simulink model "vertical_dynamics_vehicle"  (R2025a)
settings: Solver=FixedStepAuto  StartTime=0.0  StopTime=T_sim  FixedStep=T_abt  RelTol=1e-3
values from neighbouring files (symbols this model uses):
  b = 1.4    [vertical_dynamics_kf.m]
  dFh = 2000    [vertical_dynamics_kf.m]
  dFv = 1500    [vertical_dynamics_kf.m]
  dPhi_0 = 0    [vertical_dynamics_kf.m]
  dR = 250    [vertical_dynamics_kf.m]
  dTheta_0 = 0    [vertical_dynamics_kf.m]
  dz1_0 = 0    [vertical_dynamics_kf.m]
  dz2_0 = 0    [vertical_dynamics_kf.m]
  dz3_0 = 0    [vertical_dynamics_kf.m]
  dz4_0 = 0    [vertical_dynamics_kf.m]
  dz5_0 = 0    [vertical_dynamics_kf.m]
  Jphi = 500    [vertical_dynamics_kf.m]
  Jtheta = 2000    [vertical_dynamics_kf.m]
  kFh = 2200    [vertical_dynamics_kf.m]
  kFv = 2500    [vertical_dynamics_kf.m]
  kR = 100000    [vertical_dynamics_kf.m]
  lh = 1.8    [vertical_dynamics_kf.m]
  lv = 1.9    [vertical_dynamics_kf.m]
  m1 = 50    [vertical_dynamics_kf.m]
  m2 = 50    [vertical_dynamics_kf.m]
  m3 = 50    [vertical_dynamics_kf.m]
  m4 = 50    [vertical_dynamics_kf.m]
  m5 = 1200    [vertical_dynamics_kf.m]
  P_0 = Q    [vertical_dynamics_kf.m]
  Phi_0 = 0    [vertical_dynamics_kf.m]
  Q = diag([sigma_z^2,sigma_z^2,sigma_z^2,sigma_z^2,sigma_z^2,sigma_phi^2,sigma_theta^2,    sigma_dz^2,sigma_dz^2,sigma_dz^2,sigma_dz^2,sigma_dz^2,sigma_dphi^2,sigma_dtheta^2 ])*T_abt^2    [vertical_dynamics_kf.m]
  R = diag([sigma_mz^2,sigma_mz^2,sigma_mz^2,sigma_mz^2,sigma_mz^2,sigma_mphi^2,sigma_mtheta^2])    [vertical_dynamics_kf.m]
  seed = randi(1000,3,1)    [vertical_dynamics_kf.m]
  sigma_dphi = 1.6    [vertical_dynamics_kf.m]
  sigma_dtheta = 1.3    [vertical_dynamics_kf.m]
  sigma_dz = 1.1    [vertical_dynamics_kf.m]
  sigma_mphi = 0.2    [vertical_dynamics_kf.m]
  sigma_mtheta = 0.1    [vertical_dynamics_kf.m]
  sigma_mz = 0.1    [vertical_dynamics_kf.m]
  sigma_phi = 1.2    [vertical_dynamics_kf.m]
  sigma_theta = 1.7    [vertical_dynamics_kf.m]
  sigma_z = 1.5    [vertical_dynamics_kf.m]
  T_abt = 0.01    [vertical_dynamics_kf.m]
  Theta_0 = 0    [vertical_dynamics_kf.m]
  x_0 = [z1_0;z2_0;z3_0;z4_0;z5_0;Phi_0;Theta_0;dz1_0;dz2_0;dz3_0;dz4_0;dz5_0;dPhi_0;dTheta_0]    [vertical_dynamics_kf.m]
  z1_0 = 0    [vertical_dynamics_kf.m]
  z2_0 = 0    [vertical_dynamics_kf.m]
  z3_0 = 0    [vertical_dynamics_kf.m]
  z4_0 = 0    [vertical_dynamics_kf.m]
  z5_0 = 0    [vertical_dynamics_kf.m]
(part 1 of 2)
settings Model: Creator=Meng Lingbing  LastModifiedBy=CelestialAurora
settings DataIOCC: ReturnWorkspaceOutputs=off
settings RTWCC: GPUComputeCapability=3.5

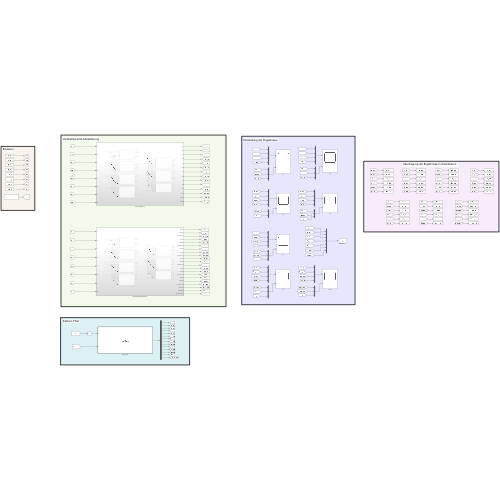
[thumbnail: Simulink's stored preview of the top-level diagram]
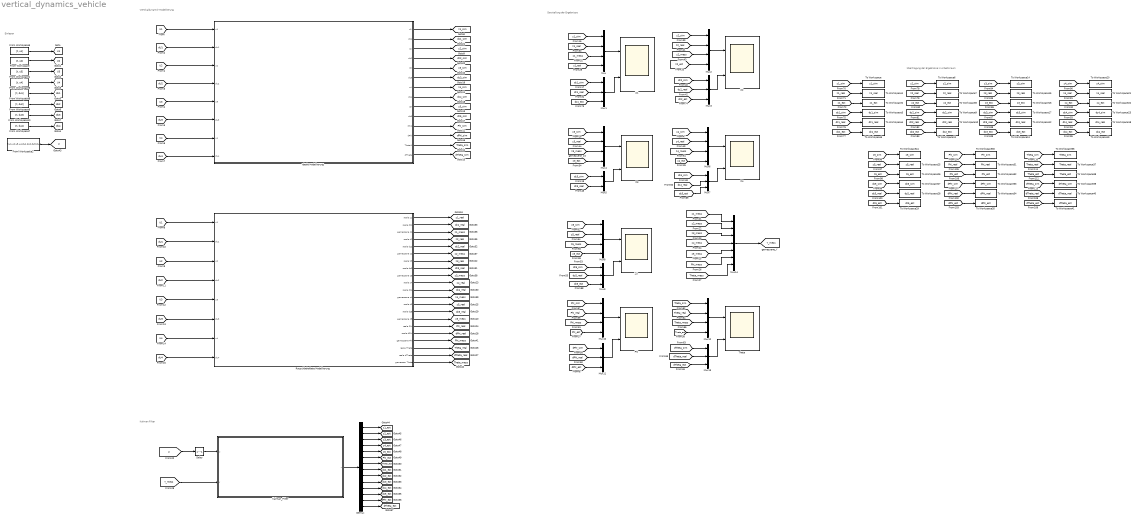
== system vertical_dynamics_vehicle ==
  note: Übertragung der Ergebnisse in Arbeitsraum
  note: Kalman Filter
  note: Einlesen
  note: Vertikaldynamik-Modellierung
  note: Darstellung der Ergebnisse
  Delay : Delay  DelayLength=1  InitialCondition=0
  Demux : Demux  Outputs=14
  From Workspace : FromWorkspace  VariableName=[t, u2]
  From Workspace1 : FromWorkspace  VariableName=[t, u3]
  From Workspace10 : FromWorkspace  VariableName=[t, du3]
  From Workspace2 : FromWorkspace  VariableName=[t,u1,u2,u3,u4,du1,du2,du3,du4]
  From Workspace5 : FromWorkspace  VariableName=[t, u1]
  From Workspace6 : FromWorkspace  VariableName=[t, u4]
  From Workspace7 : FromWorkspace  VariableName=[t, du4]
  From Workspace8 : FromWorkspace  VariableName=[t, du1]
  From Workspace9 : FromWorkspace  VariableName=[t, du2]
  Ideale Modellierung : Subsystem
  Kalman_Filter : MATLAB Function  TreatAsAtomicUnit=on
  Mux{,2,4,6,8,10,12} (7 alike) : Mux
  Mux{1,3,7,9,11,13} (6 alike) : Mux  Inputs=3
  Mux14 : Mux  Inputs=7
  Mux5 : Mux  Inputs=2
  Phi : Scope  NumInputPorts=2
      settings: Title=Phi  ActiveDisplayYMinimum=-0.7996543826921555  ActiveDisplayYMaximum=0.79993168814279936  DataLoggingVariableName=ScopeData5
  Rauschbehaftete Modellierung : Subsystem
  Theta : Scope  NumInputPorts=2
      settings: Title=Theta  ActiveDisplayYMinimum=-0.43128  ActiveDisplayYMaximum=0.39189  DataLoggingVariableName=ScopeData6
  To Workspace : ToWorkspace  VariableName=z1_sim  SampleTime=-1
      settings: Save2DSignal=2-D array (concatenate along first dimension)
  To Workspace1 : ToWorkspace  VariableName=z1_real  SampleTime=-1
      settings: Save2DSignal=2-D array (concatenate along first dimension)
  To Workspace10 : ToWorkspace  VariableName=dz2_real  SampleTime=-1
      settings: Save2DSignal=2-D array (concatenate along first dimension)
  To Workspace11 : ToWorkspace  VariableName=dz2_est  SampleTime=-1
      settings: Save2DSignal=2-D array (concatenate along first dimension)
  To Workspace12 : ToWorkspace  VariableName=dz3_real  SampleTime=-1
      settings: Save2DSignal=2-D array (concatenate along first dimension)
  To Workspace13 : ToWorkspace  VariableName=dz3_est  SampleTime=-1
      settings: Save2DSignal=2-D array (concatenate along first dimension)
  To Workspace14 : ToWorkspace  VariableName=z3_sim  SampleTime=-1
      settings: Save2DSignal=2-D array (concatenate along first dimension)
  To Workspace15 : ToWorkspace  VariableName=z3_real  SampleTime=-1
      settings: Save2DSignal=2-D array (concatenate along first dimension)
  To Workspace16 : ToWorkspace  VariableName=z3_est  SampleTime=-1
      settings: Save2DSignal=2-D array (concatenate along first dimension)
  To Workspace17 : ToWorkspace  VariableName=dz3_sim  SampleTime=-1
      settings: Save2DSignal=2-D array (concatenate along first dimension)
  To Workspace18 : ToWorkspace  VariableName=dz4_real  SampleTime=-1
      settings: Save2DSignal=2-D array (concatenate along first dimension)
  To Workspace19 : ToWorkspace  VariableName=dz4_est  SampleTime=-1
      settings: Save2DSignal=2-D array (concatenate along first dimension)
  To Workspace2 : ToWorkspace  VariableName=z1_est  SampleTime=-1
      settings: Save2DSignal=2-D array (concatenate along first dimension)
  To Workspace20 : ToWorkspace  VariableName=z4_sim  SampleTime=-1
      settings: Save2DSignal=2-D array (concatenate along first dimension)
  To Workspace21 : ToWorkspace  VariableName=z4_real  SampleTime=-1
      settings: Save2DSignal=2-D array (concatenate along first dimension)
  To Workspace22 : ToWorkspace  VariableName=z4_est  SampleTime=-1
      settings: Save2DSignal=2-D array (concatenate along first dimension)
  To Workspace23 : ToWorkspace  VariableName=dz4_sim  SampleTime=-1
      settings: Save2DSignal=2-D array (concatenate along first dimension)
  To Workspace24 : ToWorkspace  VariableName=z5_sim  SampleTime=-1
      settings: Save2DSignal=2-D array (concatenate along first dimension)
  To Workspace25 : ToWorkspace  VariableName=z5_real  SampleTime=-1
      settings: Save2DSignal=2-D array (concatenate along first dimension)
  To Workspace26 : ToWorkspace  VariableName=z5_est  SampleTime=-1
      settings: Save2DSignal=2-D array (concatenate along first dimension)
  To Workspace27 : ToWorkspace  VariableName=dz5_sim  SampleTime=-1
      settings: Save2DSignal=2-D array (concatenate along first dimension)
  To Workspace28 : ToWorkspace  VariableName=dz5_real  SampleTime=-1
      settings: Save2DSignal=2-D array (concatenate along first dimension)
  To Workspace29 : ToWorkspace  VariableName=dz5_est  SampleTime=-1
      settings: Save2DSignal=2-D array (concatenate along first dimension)
  To Workspace3 : ToWorkspace  VariableName=dz1_sim  SampleTime=-1
      settings: Save2DSignal=2-D array (concatenate along first dimension)
  To Workspace30 : ToWorkspace  VariableName=Phi_sim  SampleTime=-1
      settings: Save2DSignal=2-D array (concatenate along first dimension)
  To Workspace31 : ToWorkspace  VariableName=Phi_real  SampleTime=-1
      settings: Save2DSignal=2-D array (concatenate along first dimension)
  To Workspace32 : ToWorkspace  VariableName=Phi_est  SampleTime=-1
      settings: Save2DSignal=2-D array (concatenate along first dimension)
  To Workspace33 : ToWorkspace  VariableName=dPhi_sim  SampleTime=-1
      settings: Save2DSignal=2-D array (concatenate along first dimension)
  To Workspace34 : ToWorkspace  VariableName=dPhi_real  SampleTime=-1
      settings: Save2DSignal=2-D array (concatenate along first dimension)
  To Workspace35 : ToWorkspace  VariableName=dPhi_est  SampleTime=-1
      settings: Save2DSignal=2-D array (concatenate along first dimension)
  To Workspace36 : ToWorkspace  VariableName=Theta_sim  SampleTime=-1
      settings: Save2DSignal=2-D array (concatenate along first dimension)
  To Workspace37 : ToWorkspace  VariableName=Theta_real  SampleTime=-1
      settings: Save2DSignal=2-D array (concatenate along first dimension)
  To Workspace38 : ToWorkspace  VariableName=Theta_est  SampleTime=-1
      settings: Save2DSignal=2-D array (concatenate along first dimension)
  To Workspace39 : ToWorkspace  VariableName=dTheta_sim  SampleTime=-1
      settings: Save2DSignal=2-D array (concatenate along first dimension)
  To Workspace4 : ToWorkspace  VariableName=dz1_real  SampleTime=-1
      settings: Save2DSignal=2-D array (concatenate along first dimension)
  To Workspace40 : ToWorkspace  VariableName=dTheta_real  SampleTime=-1
      settings: Save2DSignal=2-D array (concatenate along first dimension)
  To Workspace41 : ToWorkspace  VariableName=dTheta_est  SampleTime=-1
      settings: Save2DSignal=2-D array (concatenate along first dimension)
  To Workspace5 : ToWorkspace  VariableName=dz1_est  SampleTime=-1
      settings: Save2DSignal=2-D array (concatenate along first dimension)
  To Workspace6 : ToWorkspace  VariableName=z2_sim  SampleTime=-1
      settings: Save2DSignal=2-D array (concatenate along first dimension)
  To Workspace7 : ToWorkspace  VariableName=z2_real  SampleTime=-1
      settings: Save2DSignal=2-D array (concatenate along first dimension)
  To Workspace8 : ToWorkspace  VariableName=z2_est  SampleTime=-1
      settings: Save2DSignal=2-D array (concatenate along first dimension)
  To Workspace9 : ToWorkspace  VariableName=dz2_sim  SampleTime=-1
      settings: Save2DSignal=2-D array (concatenate along first dimension)
  Z{1..5} (5 alike) : Scope  NumInputPorts=2
      Z1 settings: ActiveDisplayYMinimum=-0.48807654529336147  ActiveDisplayYMaximum=0.4265472667177741  DataLoggingVariableName=Z1  DataLoggingSaveFormat=Structure
      Z2 settings: ActiveDisplayYMinimum=-4.09102  ActiveDisplayYMaximum=3.79326
      Z3 settings: ActiveDisplayYMinimum=-4.04069  ActiveDisplayYMaximum=4.12549  DataLoggingVariableName=ScopeData2
      Z4 settings: ActiveDisplayYMinimum=-3.98296  ActiveDisplayYMaximum=4.0701  DataLoggingVariableName=ScopeData3
      Z5 settings: Title=Z5  ActiveDisplayYMinimum=-0.43929  ActiveDisplayYMaximum=0.39174  DataLoggingVariableName=ScopeData4
  tag scope: Phi_est=global, Phi_mess=global, Phi_real=global, Phi_sim=global, Theta_est=global, Theta_mess=global, Theta_real=global, Theta_sim=global, U1=global, U2=global, U3=global, U4=global, U=global, Y_mess=global, dPhi_est=global, dPhi_real=global, dPhi_sim=global, dTheta_est=global, dTheta_real=global, dTheta_sim=global, dU1=global, dU2=global, dU3=global, dU4=global, dz1_est=global, dz1_real=global, dz1_sim=global, dz2_est=global, dz2_real=global, dz2_sim=global, dz3_est=global, dz3_real=global, dz3_sim=global, dz4_est=global, dz4_real=global, dz4_sim=global, dz5_est=global, dz5_real=global, dz5_sim=global, z1_est=global, z1_mess=global, z1_real=global, z1_sim=global, z2_est=global, z2_mess=global, z2_real=global, z2_sim=global, z3_est=global, z3_mess=global, z3_real=global, z3_sim=global, z4_est=global, z4_mess=global, z4_real=global, z4_sim=global, z5_est=global, z5_mess=global, z5_real=global, z5_sim=global
  wires:
  From Workspace5/1 -> [U1]
  From Workspace/1 -> [U2]
  From Workspace1/1 -> [U3]
  From Workspace6/1 -> [U4]
  From Workspace7/1 -> [dU4]
  From Workspace8/1 -> [dU1]
  From Workspace9/1 -> [dU2]
  From Workspace10/1 -> [dU3]
  [U1] -> Ideale Modellierung/1(u1)
  [dU1] -> Ideale Modellierung/2(du1)
  [U2] -> Ideale Modellierung/3(u2)
  [dU2] -> Ideale Modellierung/4(du2)
  [U3] -> Ideale Modellierung/5(u3)
  [dU3] -> Ideale Modellierung/6(du3)
  [U4] -> Ideale Modellierung/7(u4)
  [dU4] -> Ideale Modellierung/8(du4)
  Ideale Modellierung/1(z1) -> [z1_sim]
  Ideale Modellierung/3(z2) -> [z2_sim]
  Ideale Modellierung/5(z3) -> [z3_sim]
  Ideale Modellierung/7(z4) -> [z4_sim]
  Ideale Modellierung/9(z5) -> [z5_sim]
  Ideale Modellierung/11(Phi1) -> [Phi_sim]
  Ideale Modellierung/13(Theta1) -> [Theta_sim]
  Ideale Modellierung/2(dz1) -> [dz1_sim]
  Ideale Modellierung/10(dz5) -> [dz5_sim]
  Ideale Modellierung/8(dz4) -> [dz4_sim]
  Ideale Modellierung/6(dz3) -> [dz3_sim]
  Ideale Modellierung/4(dz2) -> [dz2_sim]
  Ideale Modellierung/12(dPhi) -> [dPhi_sim]
  Ideale Modellierung/14(dTheta) -> [dTheta_sim]
  Rauschbehaftete Modellierung/17(reale dPhi) -> [dPhi_real]
  Rauschbehaftete Modellierung/1(reale z1) -> [z1_real]
  [dU3] -> Rauschbehaftete Modellierung/6(du3)
  [dU4] -> Rauschbehaftete Modellierung/8(du4)
  Rauschbehaftete Modellierung/13(reale z5) -> [z5_real]
  Rauschbehaftete Modellierung/7(reale z3) -> [z3_real]
  Rauschbehaftete Modellierung/19(reale Theta) -> [Theta_real]
  Rauschbehaftete Modellierung/10(reale z4) -> [z4_real]
  Rauschbehaftete Modellierung/16(reale Phi) -> [Phi_real]
  [U3] -> Rauschbehaftete Modellierung/5(u3)
  [dU2] -> Rauschbehaftete Modellierung/4(du2)
  Rauschbehaftete Modellierung/4(reale z2) -> [z2_real]
  [U1] -> Rauschbehaftete Modellierung/1(u1)
  [dU1] -> Rauschbehaftete Modellierung/2(du1)
  Rauschbehaftete Modellierung/5(reale dz2) -> [dz2_real]
  Rauschbehaftete Modellierung/8(reale dz3) -> [dz3_real]
  Rauschbehaftete Modellierung/14(reale dz5) -> [dz5_real]
  Rauschbehaftete Modellierung/11(reale dz4) -> [dz4_real]
  Rauschbehaftete Modellierung/20(reale dTheta) -> [dTheta_real]
  [U2] -> Rauschbehaftete Modellierung/3(u2)
  [U4] -> Rauschbehaftete Modellierung/7(u4)
  Rauschbehaftete Modellierung/2(reale dz1) -> [dz1_real]
  Rauschbehaftete Modellierung/3(gemessene z1) -> [z1_mess]
  Rauschbehaftete Modellierung/6(gemessene z2) -> [z2_mess]
  Rauschbehaftete Modellierung/9(gemessene z3) -> [z3_mess]
  Rauschbehaftete Modellierung/12(gemessene z4) -> [z4_mess]
  Rauschbehaftete Modellierung/15(gemessene z5) -> [z5_mess]
  Rauschbehaftete Modellierung/18(gemessene Phi) -> [Phi_mess]
  Rauschbehaftete Modellierung/21(gemessen Theta) -> [Theta_mess]
  [z1_sim] -> Mux/1
  [z1_real] -> Mux/2
  [z1_mess] -> Mux/3
  [dz1_sim] -> Mux1/1
  [dz1_real] -> Mux1/2
  Mux/1 -> Z1/1
  Mux1/1 -> Z1/2
  [z2_sim] -> Mux2/1
  [dz2_real] -> Mux3/2
  [dz2_sim] -> Mux3/1
  Mux2/1 -> Z2/1
  [z2_real] -> Mux2/2
  Mux3/1 -> Z2/2
  [z2_mess] -> Mux2/3
  [z3_sim] -> Mux4/1
  [dz3_real] -> Mux5/2
  [dz3_sim] -> Mux5/1
  Mux4/1 -> Z3/1
  [z3_real] -> Mux4/2
  Mux5/1 -> Z3/2
  [z3_mess] -> Mux4/3
  [z4_real] -> Mux6/2
  Mux6/1 -> Z4/1
  [z4_mess] -> Mux6/3
  [dz4_sim] -> Mux7/1
  [dz4_real] -> Mux7/2
  [z4_sim] -> Mux6/1
  Mux7/1 -> Z4/2
  Mux9/1 -> Z5/2
  [z5_real] -> Mux8/2
  Mux8/1 -> Z5/1
  [z5_sim] -> Mux8/1
  [dz5_sim] -> Mux9/1
  [z5_mess] -> Mux8/3
  [dz5_real] -> Mux9/2
  Mux11/1 -> Phi/2
  [Phi_real] -> Mux10/2
  Mux10/1 -> Phi/1
  [Phi_sim] -> Mux10/1
  [dPhi_sim] -> Mux11/1
  [Phi_mess] -> Mux10/3
  [dPhi_real] -> Mux11/2
  Mux13/1 -> Theta/2
  [Theta_real] -> Mux12/2
  Mux12/1 -> Theta/1
  [Theta_sim] -> Mux12/1
  [dTheta_sim] -> Mux13/1
  [Theta_mess] -> Mux12/3
  [dTheta_real] -> Mux13/2
  From Workspace2/1 -> [U]
  [U] -> Delay/1
  [z4_mess] -> Mux14/4
  [z3_mess] -> Mux14/3
  [z2_mess] -> Mux14/2
  [z1_mess] -> Mux14/1
  [z5_mess] -> Mux14/5
  [Phi_mess] -> Mux14/6
  [Theta_mess] -> Mux14/7
  Mux14/1 -> [Y_mess]
  [Y_mess] -> Kalman_Filter/2(y)
  Kalman_Filter/1(x) -> Demux/1
  Demux/1 -> [z1_est]
  Demux/2 -> [z2_est]
  Demux/3 -> [z3_est]
  Demux/4 -> [z4_est]
  Demux/5 -> [z5_est]
  Demux/6 -> [Phi_est]
  Demux/7 -> [Theta_est]
  Demux/8 -> [dz1_est]
  Demux/9 -> [dz2_est]
  Demux/10 -> [dz3_est]
  Demux/11 -> [dz4_est]
  Demux/12 -> [dz5_est]
  Demux/13 -> [dPhi_est]
  Demux/14 -> [dTheta_est]
  Delay/1 -> Kalman_Filter/1(u)
  [z1_est] -> Mux/4
  [z2_est] -> Mux2/4
  [z3_est] -> Mux4/4
  [z4_est] -> Mux6/4
  [z5_est] -> Mux8/4
  [Phi_est] -> Mux10/4
  [Theta_est] -> Mux12/4
  [dTheta_est] -> Mux13/3
  [dPhi_est] -> Mux11/3
  [dz5_est] -> Mux9/3
  [dz5_est] -> Mux7/3
  [dz1_est] -> Mux1/3
  [dz2_est] -> Mux3/3
  [z1_sim] -> To Workspace/1
  [z1_real] -> To Workspace1/1
  [z1_est] -> To Workspace2/1
  [dz1_est] -> To Workspace5/1
  [dz1_real] -> To Workspace4/1
  [dz1_sim] -> To Workspace3/1
  [dz2_est] -> To Workspace11/1
  [dz2_sim] -> To Workspace9/1
  [z2_real] -> To Workspace7/1
  [dz2_real] -> To Workspace10/1
  [z2_sim] -> To Workspace6/1
  [z2_est] -> To Workspace8/1
  [z3_est] -> To Workspace16/1
  [z3_real] -> To Workspace15/1
  [dz3_est] -> To Workspace13/1
  [z3_sim] -> To Workspace14/1
  [dz3_real] -> To Workspace12/1
  [dz3_sim] -> To Workspace17/1
  [dz4_sim] -> To Workspace23/1
  [dz4_real] -> To Workspace18/1
  [z4_sim] -> To Workspace20/1
  [dz4_est] -> To Workspace19/1
  [z4_real] -> To Workspace21/1
  [z4_est] -> To Workspace22/1
  [dz5_est] -> To Workspace29/1
  [dz5_sim] -> To Workspace27/1
  [z5_real] -> To Workspace25/1
  [dz5_real] -> To Workspace28/1
  [z5_sim] -> To Workspace24/1
  [z5_est] -> To Workspace26/1
  [Phi_sim] -> To Workspace30/1
  [dPhi_sim] -> To Workspace33/1
  [Phi_est] -> To Workspace32/1
  [dPhi_real] -> To Workspace34/1
  [Phi_real] -> To Workspace31/1
  [dPhi_est] -> To Workspace35/1
  [Theta_real] -> To Workspace37/1
  [dTheta_est] -> To Workspace41/1
  [dTheta_sim] -> To Workspace39/1
  [dTheta_real] -> To Workspace40/1
  [Theta_est] -> To Workspace38/1
  [Theta_sim] -> To Workspace36/1

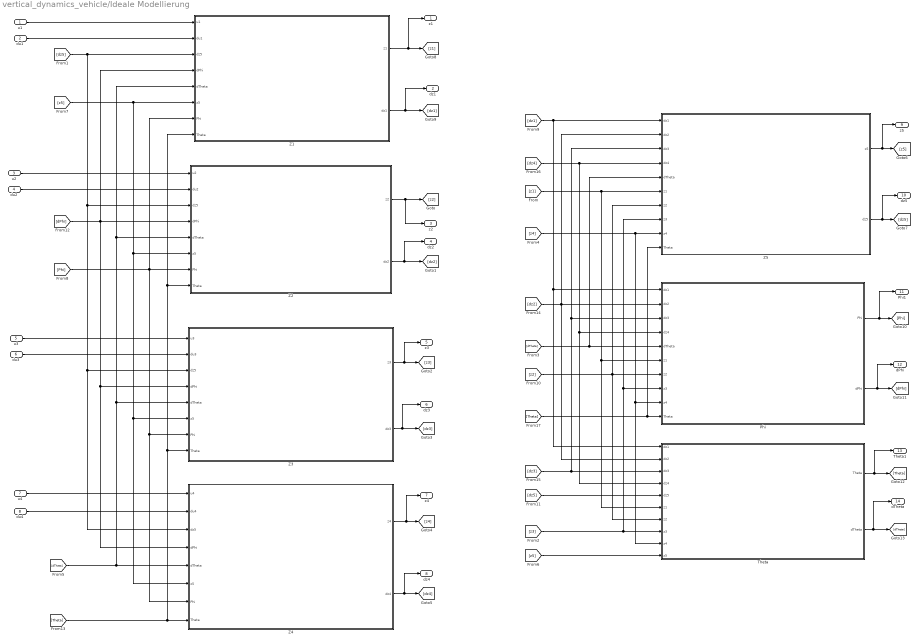
== system vertical_dynamics_vehicle/Ideale Modellierung ==
  u1 : Inport
  du1 : Inport  Port=2
  u2 : Inport  Port=3
  du2 : Inport  Port=4
  u3 : Inport  Port=5
  du3 : Inport  Port=6
  u4 : Inport  Port=7
  du4 : Inport  Port=8
  Phi : Subsystem
  Theta : Subsystem
  Z1 : Subsystem
  Z2 : Subsystem
  Z3 : Subsystem
  Z4 : Subsystem
  Z5 : Subsystem
  z1 : Outport
  dz1 : Outport  Port=2
  z2 : Outport  Port=3
  dz2 : Outport  Port=4
  z3 : Outport  Port=5
  dz3 : Outport  Port=6
  z4 : Outport  Port=7
  dz4 : Outport  Port=8
  z5 : Outport  Port=9
  dz5 : Outport  Port=10
  Phi1 : Outport  Port=11
  dPhi : Outport  Port=12
  Theta1 : Outport  Port=13
  dTheta : Outport  Port=14
  wires:
  Theta/1(Theta) -> Theta1/1, [Theta]
  Z1/1(z1) -> z1/1, [z1]
  Z1/2(dz1) -> dz1/1, [dz1]
  Z2/1(z2) -> z2/1, [z2]
  Z5/1(z5) -> [z5], z5/1
  Phi/1(Phi) -> [Phi], Phi1/1
  u1/1 -> Z1/1(u1)
  u4/1 -> Z4/1(u4)
  du4/1 -> Z4/2(du4)
  du1/1 -> Z1/2(du1)
  u2/1 -> Z2/1(u2)
  du2/1 -> Z2/2(du2)
  du3/1 -> Z3/2(du3)
  u3/1 -> Z3/1(u3)
  Z2/2(dz2) -> dz2/1, [dz2]
  Z3/1(z3) -> z3/1, [z3]
  Z3/2(dz3) -> dz3/1, [dz3]
  Z4/1(z4) -> [z4], z4/1
  Z4/2(dz4) -> dz4/1, [dz4]
  Z5/2(dz5) -> [dz5], dz5/1
  Phi/2(dPhi) -> dPhi/1, [dPhi]
  Theta/2(dTheta) -> dTheta/1, [dTheta]
  [z1] -> Z5/6(z1), Phi/6(z1), Theta/6(z1)
  [dTheta] -> Phi/5(dTheta), Z5/5(dTheta)
  [dTheta] -> Z4/5(dTheta), Z3/5(dTheta), Z2/5(dTheta), Z1/5(dTheta)
  [dz1] -> Z5/1(dz1), Phi/1(dz1), Theta/1(dz1)
  [z2] -> Phi/7(z2), Theta/7(z2), Z5/7(z2)
  [z3] -> Phi/8(z3), Z5/8(z3), Theta/8(z3)
  [dz5] -> Z1/3(dz5), Z4/3(dz5), Z3/3(dz5), Z2/3(dz5)
  [dz5] -> Theta/5(dz5)
  [dPhi] -> Z2/4(dPhi), Z3/4(dPhi), Z4/4(dPhi), Z1/4(dPhi)
  [z5] -> Z1/6(z5), Z2/6(z5), Z3/6(z5), Z4/6(z5)
  [Phi] -> Z3/7(Phi), Z4/7(Phi), Z1/7(Phi), Z2/7(Phi)
  [Theta] -> Z4/8(Theta), Z3/8(Theta), Z2/8(Theta), Z1/8(Theta)
  [dz2] -> Z5/2(dz2), Theta/2(dz2), Phi/2(dz2)
  [dz3] -> Theta/3(dz3), Phi/3(dz3), Z5/3(dz3)
  [dz4] -> Z5/4(dz4), Phi/4(dz4), Theta/4(dz4)
  [z4] -> Z5/9(z4), Phi/9(z4), Theta/9(z4)
  [Theta] -> Phi/10(Theta), Z5/10(Theta)
  [z5] -> Theta/10(z5)

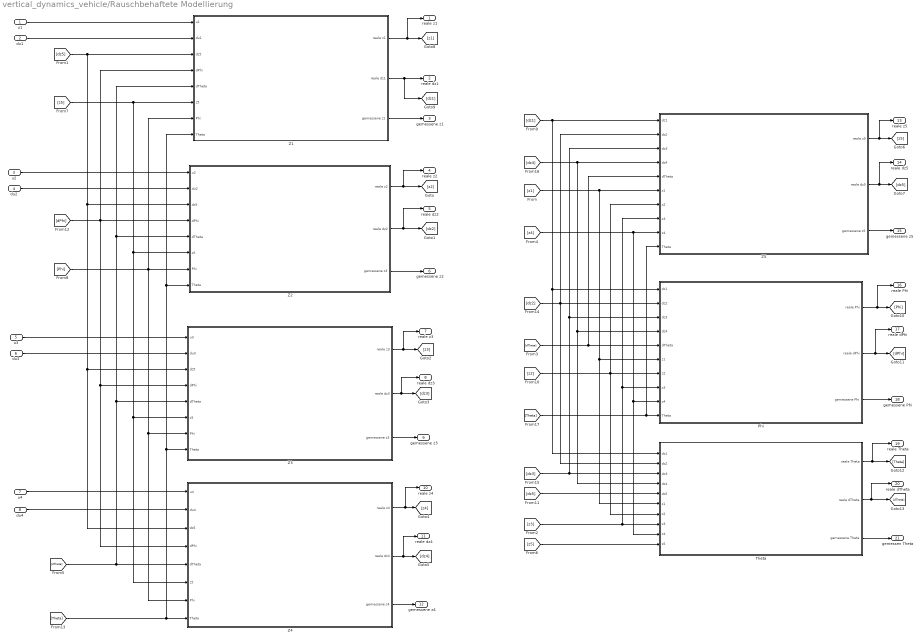
== system vertical_dynamics_vehicle/Rauschbehaftete Modellierung ==
  u1 : Inport
  du1 : Inport  Port=2
  u2 : Inport  Port=3
  du2 : Inport  Port=4
  u3 : Inport  Port=5
  du3 : Inport  Port=6
  u4 : Inport  Port=7
  du4 : Inport  Port=8
  Phi : Subsystem
  Theta : Subsystem
  Z1 : Subsystem
  Z2 : Subsystem
  Z3 : Subsystem
  Z4 : Subsystem
  Z5 : Subsystem
  reale z1 : Outport
  reale dz1 : Outport  Port=2
  gemessene z1 : Outport  Port=3
  reale z2 : Outport  Port=4
  reale dz2 : Outport  Port=5
  gemessene z2 : Outport  Port=6
  reale z3 : Outport  Port=7
  reale dz3 : Outport  Port=8
  gemessene z3 : Outport  Port=9
  reale z4 : Outport  Port=10
  reale dz4 : Outport  Port=11
  gemessene z4 : Outport  Port=12
  reale z5 : Outport  Port=13
  reale dz5 : Outport  Port=14
  gemessene z5 : Outport  Port=15
  reale Phi : Outport  Port=16
  reale dPhi : Outport  Port=17
  gemessene Phi : Outport  Port=18
  reale Theta : Outport  Port=19
  reale dTheta : Outport  Port=20
  gemessen Theta : Outport  Port=21
  wires:
  Theta/1(reale Theta) -> [Theta], reale Theta/1
  Z1/1(reale z1) -> [z1], reale z1/1
  Z1/2(reale dz1) -> [dz1], reale dz1/1
  Z2/1(reale z2) -> [z2], reale z2/1
  Z5/1(reale z5) -> [z5], reale z5/1
  Phi/1(reale Phi) -> [Phi], reale Phi/1
  u1/1 -> Z1/1(u1)
  u4/1 -> Z4/1(u4)
  du4/1 -> Z4/2(du4)
  du1/1 -> Z1/2(du1)
  u2/1 -> Z2/1(u2)
  du2/1 -> Z2/2(du2)
  du3/1 -> Z3/2(du3)
  u3/1 -> Z3/1(u3)
  Z2/2(reale dz2) -> [dz2], reale dz2/1
  Z3/1(reale z3) -> [z3], reale z3/1
  Z3/2(reale dz3) -> [dz3], reale dz3/1
  Z4/1(reale z4) -> [z4], reale z4/1
  Z4/2(reale dz4) -> [dz4], reale dz4/1
  Z5/2(reale dz5) -> [dz5], reale dz5/1
  Phi/2(reale dPhi) -> [dPhi], reale dPhi/1
  Theta/2(reale dTheta) -> [dTheta], reale dTheta/1
  [z1] -> Z5/6(z1), Phi/6(z1), Theta/6(z1)
  [dTheta] -> Phi/5(dTheta), Z5/5(dTheta)
  [dTheta] -> Z4/5(dTheta), Z3/5(dTheta), Z2/5(dTheta), Z1/5(dTheta)
  [dz1] -> Z5/1(dz1), Phi/1(dz1), Theta/1(dz1)
  [z2] -> Phi/7(z2), Theta/7(z2), Z5/7(z2)
  [z3] -> Theta/8(z3), Phi/8(z3), Z5/8(z3)
  [dz5] -> Z1/3(dz5), Z4/3(dz5), Z3/3(dz5), Z2/3(dz5)
  [dz5] -> Theta/5(dz5)
  [dPhi] -> Z2/4(dPhi), Z3/4(dPhi), Z4/4(dPhi), Z1/4(dPhi)
  [z5] -> Z1/6(z5), Z2/6(z5), Z3/6(z5), Z4/6(z5)
  [Phi] -> Z3/7(Phi), Z4/7(Phi), Z1/7(Phi), Z2/7(Phi)
  [Theta] -> Z4/8(Theta), Z3/8(Theta), Z2/8(Theta), Z1/8(Theta)
  [dz2] -> Z5/2(dz2), Theta/2(dz2), Phi/2(dz2)
  [dz3] -> Theta/3(dz3), Phi/3(dz3), Z5/3(dz3)
  [dz4] -> Z5/4(dz4), Phi/4(dz4), Theta/4(dz4)
  [z4] -> Z5/9(z4), Phi/9(z4), Theta/9(z4)
  [Theta] -> Phi/10(Theta), Z5/10(Theta)
  [z5] -> Theta/10(z5)
  Z1/3(gemessene z1) -> gemessene z1/1
  Z2/3(gemessene z3) -> gemessene z2/1
  Z3/3(gemessene z3) -> gemessene z3/1
  Z4/3(gemessene z4) -> gemessene z4/1
  Z5/3(gemessene z5) -> gemessene z5/1
  Phi/3(gemessene Phi) -> gemessene Phi/1
  Theta/3(gemessene Theta) -> gemessen Theta/1

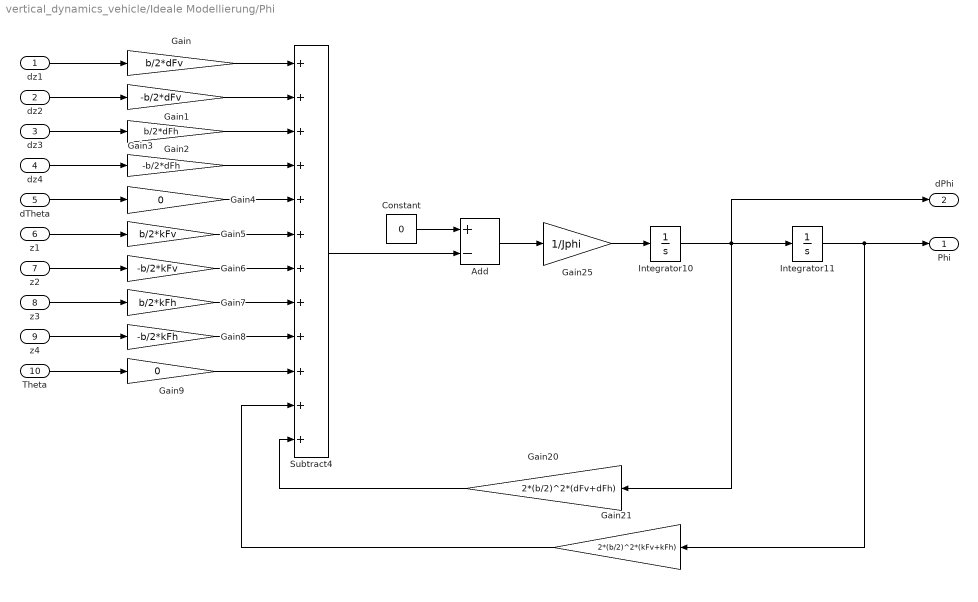
== system vertical_dynamics_vehicle/Ideale Modellierung/Phi ==
  dz1 : Inport
  dz2 : Inport  Port=2
  dz3 : Inport  Port=3
  dz4 : Inport  Port=4
  dTheta : Inport  Port=5
  z1 : Inport  Port=6
  z2 : Inport  Port=7
  z3 : Inport  Port=8
  z4 : Inport  Port=9
  Theta : Inport  Port=10
  Add : Sum  Inputs=+-
  Constant : Constant  Value=0
  Gain : Gain  Gain=b/2*dFv
  Gain1 : Gain  Gain=-b/2*dFv
  Gain2 : Gain  Gain=b/2*dFh
  Gain20 : Gain  Gain=2*(b/2)^2*(dFv+dFh)
  Gain21 : Gain  Gain=2*(b/2)^2*(kFv+kFh)
  Gain25 : Gain  Gain=1/Jphi
  Gain3 : Gain  Gain=-b/2*dFh
  Gain4 : Gain  Gain=0
  Gain5 : Gain  Gain=b/2*kFv
  Gain6 : Gain  Gain=-b/2*kFv
  Gain7 : Gain  Gain=b/2*kFh
  Gain8 : Gain  Gain=-b/2*kFh
  Gain9 : Gain  Gain=0
  Integrator10 : Integrator  InitialCondition=dPhi_0
  Integrator11 : Integrator  InitialCondition=Phi_0
  Subtract4 : Sum  Inputs=++++++++++++
  Phi : Outport
  dPhi : Outport  Port=2
  wires:
  Integrator11/1 -> Phi/1, Gain21/1
  Integrator10/1 -> Integrator11/1, dPhi/1, Gain20/1
  Gain25/1 -> Integrator10/1
  dz1/1 -> Gain/1
  Gain2/1 -> Subtract4/3
  z1/1 -> Gain5/1
  Gain9/1 -> Subtract4/10
  z3/1 -> Gain7/1
  Theta/1 -> Gain9/1
  Gain4/1 -> Subtract4/5
  Gain1/1 -> Subtract4/2
  dz2/1 -> Gain1/1
  Gain8/1 -> Subtract4/9
  dTheta/1 -> Gain4/1
  z4/1 -> Gain8/1
  Gain5/1 -> Subtract4/6
  Gain/1 -> Subtract4/1
  Gain6/1 -> Subtract4/7
  z2/1 -> Gain6/1
  dz4/1 -> Gain3/1
  Gain3/1 -> Subtract4/4
  Gain7/1 -> Subtract4/8
  dz3/1 -> Gain2/1
  Gain20/1 -> Subtract4/12
  Gain21/1 -> Subtract4/11
  Constant/1 -> Add/1
  Add/1 -> Gain25/1
  Subtract4/1 -> Add/2

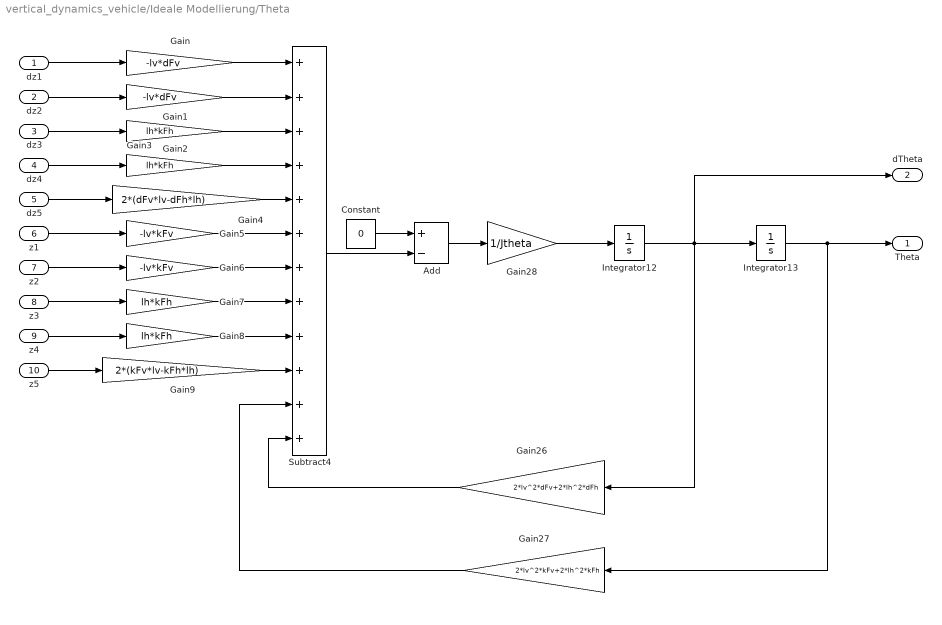
== system vertical_dynamics_vehicle/Ideale Modellierung/Theta ==
  dz1 : Inport
  dz2 : Inport  Port=2
  dz3 : Inport  Port=3
  dz4 : Inport  Port=4
  dz5 : Inport  Port=5
  z1 : Inport  Port=6
  z2 : Inport  Port=7
  z3 : Inport  Port=8
  z4 : Inport  Port=9
  z5 : Inport  Port=10
  Add : Sum  Inputs=+-
  Constant : Constant  Value=0
  Gain : Gain  Gain=-lv*dFv
  Gain1 : Gain  Gain=-lv*dFv
  Gain{2..3,7..8} (4 alike) : Gain  Gain=lh*kFh
  Gain26 : Gain  Gain=2*lv^2*dFv+2*lh^2*dFh
  Gain27 : Gain  Gain=2*lv^2*kFv+2*lh^2*kFh
  Gain28 : Gain  Gain=1/Jtheta
  Gain4 : Gain  Gain=2*(dFv*lv-dFh*lh)
  Gain5 : Gain  Gain=-lv*kFv
  Gain6 : Gain  Gain=-lv*kFv
  Gain9 : Gain  Gain=2*(kFv*lv-kFh*lh)
  Integrator12 : Integrator  InitialCondition=dTheta_0
  Integrator13 : Integrator  InitialCondition=Theta_0
  Subtract4 : Sum  Inputs=++++++++++++
  Theta : Outport
  dTheta : Outport  Port=2
  wires:
  Integrator12/1 -> Integrator13/1, dTheta/1, Gain26/1
  Integrator13/1 -> Theta/1, Gain27/1
  Gain28/1 -> Integrator12/1
  dz4/1 -> Gain3/1
  dz3/1 -> Gain2/1
  Gain7/1 -> Subtract4/8
  Gain3/1 -> Subtract4/4
  Gain/1 -> Subtract4/1
  Gain5/1 -> Subtract4/6
  dz5/1 -> Gain4/1
  Gain6/1 -> Subtract4/7
  Gain4/1 -> Subtract4/5
  Gain1/1 -> Subtract4/2
  dz2/1 -> Gain1/1
  z5/1 -> Gain9/1
  z3/1 -> Gain7/1
  dz1/1 -> Gain/1
  Gain8/1 -> Subtract4/9
  Gain9/1 -> Subtract4/10
  z1/1 -> Gain5/1
  Gain2/1 -> Subtract4/3
  z4/1 -> Gain8/1
  z2/1 -> Gain6/1
  Gain26/1 -> Subtract4/12
  Gain27/1 -> Subtract4/11
  Subtract4/1 -> Add/2
  Add/1 -> Gain28/1
  Constant/1 -> Add/1

== system vertical_dynamics_vehicle/Ideale Modellierung/Z1 ==
  u1 : Inport
  du1 : Inport  Port=2
  dz5 : Inport  Port=3
  dPhi : Inport  Port=4
  dTheta : Inport  Port=5
  z5 : Inport  Port=6
  Phi : Inport  Port=7
  Theta : Inport  Port=8
  Add : Sum
  Add1 : Sum  Inputs=8
  Add2 : Sum  Inputs=+-
  Gain : Gain  Gain=kR
  Gain1 : Gain  Gain=dR
  Gain2 : Gain  Gain=dR+dFv
  Gain29 : Gain  Gain=-dFv
  Gain3 : Gain  Gain=kR+kFv
  Gain30 : Gain  Gain=b/2*dFv
  Gain32 : Gain  Gain=-kFv
  Gain33 : Gain  Gain=b/2*kFv
  Gain34 : Gain  Gain=-lv*dFv
  Gain4 : Gain  Gain=1/m1
  Gain5 : Gain  Gain=-lv*kFv
  Integrator : Integrator  InitialCondition=dz1_0
  Integrator1 : Integrator  InitialCondition=z1_0
  z1 : Outport
  dz1 : Outport  Port=2
  wires:
  Add2/1 -> Gain4/1
  Gain1/1 -> Add/2
  Integrator/1 -> Integrator1/1, dz1/1, Gain2/1
  Gain2/1 -> Add1/1
  Add/1 -> Add2/1
  Gain/1 -> Add/1
  Gain4/1 -> Integrator/1
  Phi/1 -> Gain33/1
  Gain34/1 -> Add1/7
  Gain32/1 -> Add1/5
  Gain3/1 -> Add1/2
  Gain33/1 -> Add1/6
  u1/1 -> Gain/1
  du1/1 -> Gain1/1
  dTheta/1 -> Gain34/1
  z5/1 -> Gain32/1
  dz5/1 -> Gain29/1
  Gain29/1 -> Add1/3
  Add1/1 -> Add2/2
  Gain30/1 -> Add1/4
  dPhi/1 -> Gain30/1
  Theta/1 -> Gain5/1
  Gain5/1 -> Add1/8
  Integrator1/1 -> Gain3/1, z1/1

== system vertical_dynamics_vehicle/Ideale Modellierung/Z2 ==
  u2 : Inport
  du2 : Inport  Port=2
  dz5 : Inport  Port=3
  dPhi : Inport  Port=4
  dTheta : Inport  Port=5
  z5 : Inport  Port=6
  Phi : Inport  Port=7
  Theta : Inport  Port=8
  Add : Sum  Inputs=+-
  Add1 : Sum
  Add2 : Sum  Inputs=8
  Gain1 : Gain  Gain=-lv*kFv
  Gain29 : Gain  Gain=-dFv
  Gain30 : Gain  Gain=-b/2*dFv
  Gain32 : Gain  Gain=-kFv
  Gain33 : Gain  Gain=-b/2*kFv
  Gain34 : Gain  Gain=-lv*dFv
  Gain5 : Gain  Gain=kR
  Gain6 : Gain  Gain=dR
  Gain7 : Gain  Gain=dR+dFv
  Gain8 : Gain  Gain=kR+kFv
  Gain9 : Gain  Gain=1/m2
  Integrator2 : Integrator  InitialCondition=dz2_0
  Integrator3 : Integrator  InitialCondition=z2_0
  z2 : Outport
  dz2 : Outport  Port=2
  wires:
  Integrator2/1 -> Integrator3/1, dz2/1, Gain7/1
  Gain5/1 -> Add1/1
  du2/1 -> Gain6/1
  Integrator3/1 -> z2/1, Gain8/1
  u2/1 -> Gain5/1
  Gain9/1 -> Integrator2/1
  Gain6/1 -> Add1/2
  Gain30/1 -> Add2/4
  Gain1/1 -> Add2/8
  Theta/1 -> Gain1/1
  dPhi/1 -> Gain30/1
  Gain29/1 -> Add2/3
  Gain8/1 -> Add2/2
  Gain34/1 -> Add2/7
  dz5/1 -> Gain29/1
  Add2/1 -> Add/2
  dTheta/1 -> Gain34/1
  Gain32/1 -> Add2/5
  z5/1 -> Gain32/1
  Gain33/1 -> Add2/6
  Gain7/1 -> Add2/1
  Phi/1 -> Gain33/1
  Add1/1 -> Add/1
  Add/1 -> Gain9/1

== system vertical_dynamics_vehicle/Ideale Modellierung/Z3 ==
  u3 : Inport
  du3 : Inport  Port=2
  dz5 : Inport  Port=3
  dPhi : Inport  Port=4
  dTheta : Inport  Port=5
  z5 : Inport  Port=6
  Phi : Inport  Port=7
  Theta : Inport  Port=8
  Add1 : Sum  Inputs=8
  Add2 : Sum
  Gain1 : Gain  Gain=lh*kFh
  Gain10 : Gain  Gain=kR
  Gain11 : Gain  Gain=dR
  Gain12 : Gain  Gain=dR+dFh
  Gain13 : Gain  Gain=kR+kFh
  Gain14 : Gain  Gain=1/m3
  Gain29 : Gain  Gain=-dFh
  Gain30 : Gain  Gain=b/2*dFh
  Gain32 : Gain  Gain=-kFh
  Gain33 : Gain  Gain=b/2*kFh
  Gain34 : Gain  Gain=lh*dFh
  Integrator4 : Integrator  InitialCondition=dz3_0
  Integrator5 : Integrator  InitialCondition=z3_0
  Subtract2 : Sum  Inputs=+-
  z3 : Outport
  dz3 : Outport  Port=2
  wires:
  Gain10/1 -> Add2/1
  Add2/1 -> Subtract2/1
  Integrator4/1 -> Integrator5/1, dz3/1, Gain12/1
  Integrator5/1 -> z3/1, Gain13/1
  Gain11/1 -> Add2/2
  Gain14/1 -> Integrator4/1
  Subtract2/1 -> Gain14/1
  du3/1 -> Gain11/1
  u3/1 -> Gain10/1
  Add1/1 -> Subtract2/2
  Gain34/1 -> Add1/5
  Gain32/1 -> Add1/6
  dz5/1 -> Gain29/1
  dPhi/1 -> Gain30/1
  Theta/1 -> Gain1/1
  Gain29/1 -> Add1/3
  Gain30/1 -> Add1/4
  Gain33/1 -> Add1/7
  Gain1/1 -> Add1/8
  Gain12/1 -> Add1/1
  Gain13/1 -> Add1/2
  Phi/1 -> Gain33/1
  z5/1 -> Gain32/1
  dTheta/1 -> Gain34/1

== system vertical_dynamics_vehicle/Ideale Modellierung/Z4 ==
  u4 : Inport
  du4 : Inport  Port=2
  dz5 : Inport  Port=3
  dPhi : Inport  Port=4
  dTheta : Inport  Port=5
  z5 : Inport  Port=6
  Phi : Inport  Port=7
  Theta : Inport  Port=8
  Add1 : Sum  Inputs=8
  Add3 : Sum
  Gain1 : Gain  Gain=lh*kFh
  Gain15 : Gain  Gain=kR
  Gain16 : Gain  Gain=dR
  Gain17 : Gain  Gain=dR+dFh
  Gain18 : Gain  Gain=kR+kFh
  Gain19 : Gain  Gain=1/m4
  Gain29 : Gain  Gain=-dFh
  Gain30 : Gain  Gain=-b/2*dFh
  Gain32 : Gain  Gain=-kFh
  Gain33 : Gain  Gain=-b/2*kFh
  Gain34 : Gain  Gain=lh*dFh
  Integrator6 : Integrator  InitialCondition=dz4_0
  Integrator7 : Integrator  InitialCondition=z4_0
  Subtract3 : Sum  Inputs=+-
  z4 : Outport
  dz4 : Outport  Port=2
  wires:
  Gain16/1 -> Add3/2
  Gain17/1 -> Add1/1
  Gain15/1 -> Add3/1
  Gain19/1 -> Integrator6/1
  Add3/1 -> Subtract3/1
  Integrator7/1 -> z4/1, Gain18/1
  Integrator6/1 -> dz4/1, Gain17/1, Integrator7/1
  Subtract3/1 -> Gain19/1
  du4/1 -> Gain16/1
  u4/1 -> Gain15/1
  Add1/1 -> Subtract3/2
  Phi/1 -> Gain33/1
  z5/1 -> Gain32/1
  dTheta/1 -> Gain34/1
  Gain33/1 -> Add1/7
  dz5/1 -> Gain29/1
  Gain32/1 -> Add1/6
  Gain34/1 -> Add1/5
  Gain29/1 -> Add1/3
  Gain1/1 -> Add1/8
  dPhi/1 -> Gain30/1
  Theta/1 -> Gain1/1
  Gain30/1 -> Add1/4
  Gain18/1 -> Add1/2

== system vertical_dynamics_vehicle/Ideale Modellierung/Z5 ==
  dz1 : Inport
  dz2 : Inport  Port=2
  dz3 : Inport  Port=3
  dz4 : Inport  Port=4
  dTheta : Inport  Port=5
  z1 : Inport  Port=6
  z2 : Inport  Port=7
  z3 : Inport  Port=8
  z4 : Inport  Port=9
  Theta : Inport  Port=10
  Add : Sum  Inputs=+-
  Constant : Constant  Value=0
  Gain : Gain  Gain=-dFv
  Gain1 : Gain  Gain=-dFv
  Gain2 : Gain  Gain=-dFh
  Gain22 : Gain  Gain=2*dFv+2*dFh
  Gain23 : Gain  Gain=2*kFv+2*kFh
  Gain24 : Gain  Gain=1/m5
  Gain3 : Gain  Gain=-dFh
  Gain4 : Gain  Gain=2*(dFv*lv-dFh*lh)
  Gain5 : Gain  Gain=-kFv
  Gain6 : Gain  Gain=-kFv
  Gain7 : Gain  Gain=-kFh
  Gain8 : Gain  Gain=-kFh
  Gain9 : Gain  Gain=2*(kFv*lv-kFh*lh)
  Integrator8 : Integrator  InitialCondition=dz5_0
  Integrator9 : Integrator  InitialCondition=z5_0
  Subtract4 : Sum  Inputs=++++++++++++
  z5 : Outport
  dz5 : Outport  Port=2
  wires:
  Integrator8/1 -> Integrator9/1, dz5/1, Gain22/1
  Subtract4/1 -> Add/2
  Integrator9/1 -> z5/1, Gain23/1
  Gain24/1 -> Integrator8/1
  dz1/1 -> Gain/1
  Gain/1 -> Subtract4/1
  Gain1/1 -> Subtract4/2
  dz2/1 -> Gain1/1
  dz3/1 -> Gain2/1
  Gain2/1 -> Subtract4/3
  Gain3/1 -> Subtract4/4
  dz4/1 -> Gain3/1
  Gain22/1 -> Subtract4/12
  Gain4/1 -> Subtract4/5
  dTheta/1 -> Gain4/1
  Gain5/1 -> Subtract4/6
  z1/1 -> Gain5/1
  z2/1 -> Gain6/1
  Gain6/1 -> Subtract4/7
  z3/1 -> Gain7/1
  Gain7/1 -> Subtract4/8
  z4/1 -> Gain8/1
  Gain8/1 -> Subtract4/9
  Gain23/1 -> Subtract4/11
  Gain9/1 -> Subtract4/10
  Theta/1 -> Gain9/1
  Add/1 -> Gain24/1
  Constant/1 -> Add/1

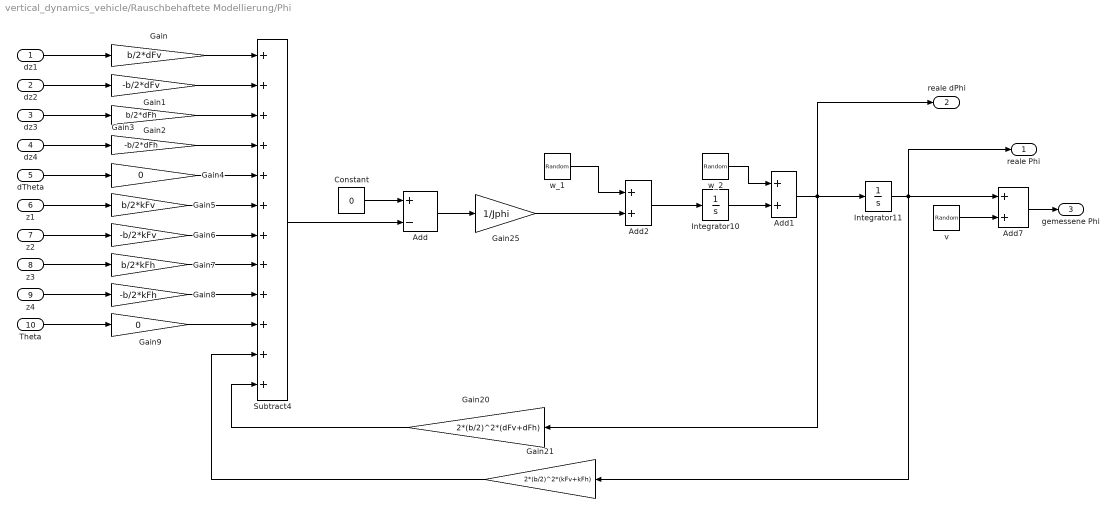
== system vertical_dynamics_vehicle/Rauschbehaftete Modellierung/Phi ==
  dz1 : Inport
  dz2 : Inport  Port=2
  dz3 : Inport  Port=3
  dz4 : Inport  Port=4
  dTheta : Inport  Port=5
  z1 : Inport  Port=6
  z2 : Inport  Port=7
  z3 : Inport  Port=8
  z4 : Inport  Port=9
  Theta : Inport  Port=10
  Add : Sum  Inputs=+-
  Add1 : Sum
  Add2 : Sum
  Add7 : Sum
  Constant : Constant  Value=0
  Gain : Gain  Gain=b/2*dFv
  Gain1 : Gain  Gain=-b/2*dFv
  Gain2 : Gain  Gain=b/2*dFh
  Gain20 : Gain  Gain=2*(b/2)^2*(dFv+dFh)
  Gain21 : Gain  Gain=2*(b/2)^2*(kFv+kFh)
  Gain25 : Gain  Gain=1/Jphi
  Gain3 : Gain  Gain=-b/2*dFh
  Gain4 : Gain  Gain=0
  Gain5 : Gain  Gain=b/2*kFv
  Gain6 : Gain  Gain=-b/2*kFv
  Gain7 : Gain  Gain=b/2*kFh
  Gain8 : Gain  Gain=-b/2*kFh
  Gain9 : Gain  Gain=0
  Integrator10 : Integrator  InitialCondition=dPhi_0
  Integrator11 : Integrator  InitialCondition=Phi_0
  Subtract4 : Sum  Inputs=++++++++++++
  v : RandomNumber  Variance=sigma_mphi^2  Seed=seed(3,1)  SampleTime=T_abt
  w_1 : RandomNumber  Variance=sigma_dphi^2  Seed=seed(1,1)  SampleTime=T_abt
  w_2 : RandomNumber  Variance=sigma_phi^2  Seed=seed(2,1)  SampleTime=T_abt
  reale Phi : Outport
  reale dPhi : Outport  Port=2
  gemessene Phi : Outport  Port=3
  wires:
  dz1/1 -> Gain/1
  Gain2/1 -> Subtract4/3
  z1/1 -> Gain5/1
  Gain9/1 -> Subtract4/10
  z3/1 -> Gain7/1
  Theta/1 -> Gain9/1
  Gain4/1 -> Subtract4/5
  Gain1/1 -> Subtract4/2
  dz2/1 -> Gain1/1
  Gain8/1 -> Subtract4/9
  dTheta/1 -> Gain4/1
  z4/1 -> Gain8/1
  Gain5/1 -> Subtract4/6
  Gain/1 -> Subtract4/1
  Gain6/1 -> Subtract4/7
  z2/1 -> Gain6/1
  dz4/1 -> Gain3/1
  Gain3/1 -> Subtract4/4
  Gain7/1 -> Subtract4/8
  dz3/1 -> Gain2/1
  Gain20/1 -> Subtract4/12
  Gain21/1 -> Subtract4/11
  Constant/1 -> Add/1
  Add/1 -> Gain25/1
  Subtract4/1 -> Add/2
  w_1/1 -> Add2/1
  w_2/1 -> Add1/1
  Gain25/1 -> Add2/2
  Add2/1 -> Integrator10/1
  Integrator10/1 -> Add1/2
  Add1/1 -> Integrator11/1, reale dPhi/1, Gain20/1
  v/1 -> Add7/2
  Add7/1 -> gemessene Phi/1
  Integrator11/1 -> Add7/1, Gain21/1, reale Phi/1

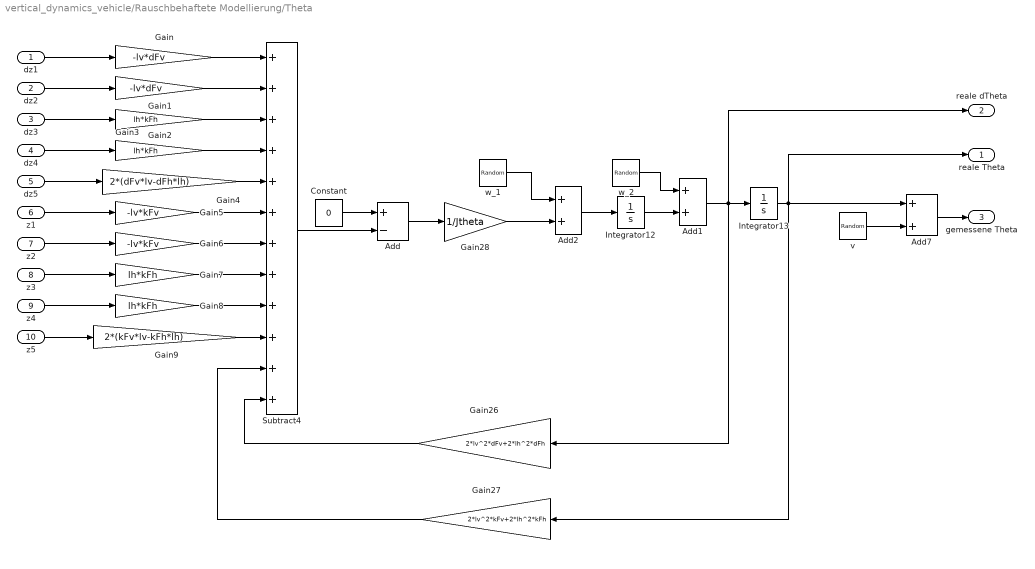
== system vertical_dynamics_vehicle/Rauschbehaftete Modellierung/Theta ==
  dz1 : Inport
  dz2 : Inport  Port=2
  dz3 : Inport  Port=3
  dz4 : Inport  Port=4
  dz5 : Inport  Port=5
  z1 : Inport  Port=6
  z2 : Inport  Port=7
  z3 : Inport  Port=8
  z4 : Inport  Port=9
  z5 : Inport  Port=10
  Add : Sum  Inputs=+-
  Add1 : Sum
  Add2 : Sum
  Add7 : Sum
  Constant : Constant  Value=0
  Gain : Gain  Gain=-lv*dFv
  Gain1 : Gain  Gain=-lv*dFv
  Gain{2..3,7..8} (4 alike) : Gain  Gain=lh*kFh
  Gain26 : Gain  Gain=2*lv^2*dFv+2*lh^2*dFh
  Gain27 : Gain  Gain=2*lv^2*kFv+2*lh^2*kFh
  Gain28 : Gain  Gain=1/Jtheta
  Gain4 : Gain  Gain=2*(dFv*lv-dFh*lh)
  Gain5 : Gain  Gain=-lv*kFv
  Gain6 : Gain  Gain=-lv*kFv
  Gain9 : Gain  Gain=2*(kFv*lv-kFh*lh)
  Integrator12 : Integrator  InitialCondition=dTheta_0
  Integrator13 : Integrator  InitialCondition=Theta_0
  Subtract4 : Sum  Inputs=++++++++++++
  v : RandomNumber  Variance=sigma_mtheta^2  Seed=seed(3,1)  SampleTime=T_abt
  w_1 : RandomNumber  Variance=sigma_dtheta^2  Seed=seed(1,1)  SampleTime=T_abt
  w_2 : RandomNumber  Variance=sigma_theta^2  Seed=seed(2,1)  SampleTime=T_abt
  reale Theta : Outport
  reale dTheta : Outport  Port=2
  gemessene Theta : Outport  Port=3
  wires:
  dz4/1 -> Gain3/1
  dz3/1 -> Gain2/1
  Gain7/1 -> Subtract4/8
  Gain3/1 -> Subtract4/4
  Gain/1 -> Subtract4/1
  Gain5/1 -> Subtract4/6
  dz5/1 -> Gain4/1
  Gain6/1 -> Subtract4/7
  Gain4/1 -> Subtract4/5
  Gain1/1 -> Subtract4/2
  dz2/1 -> Gain1/1
  z5/1 -> Gain9/1
  z3/1 -> Gain7/1
  dz1/1 -> Gain/1
  Gain8/1 -> Subtract4/9
  Gain9/1 -> Subtract4/10
  z1/1 -> Gain5/1
  Gain2/1 -> Subtract4/3
  z4/1 -> Gain8/1
  z2/1 -> Gain6/1
  Gain26/1 -> Subtract4/12
  Gain27/1 -> Subtract4/11
  Subtract4/1 -> Add/2
  Add/1 -> Gain28/1
  Constant/1 -> Add/1
  Add7/1 -> gemessene Theta/1
  v/1 -> Add7/2
  Integrator13/1 -> Gain27/1, Add7/1, reale Theta/1
  w_1/1 -> Add2/1
  w_2/1 -> Add1/1
  Gain28/1 -> Add2/2
  Add2/1 -> Integrator12/1
  Integrator12/1 -> Add1/2
  Add1/1 -> Gain26/1, reale dTheta/1, Integrator13/1

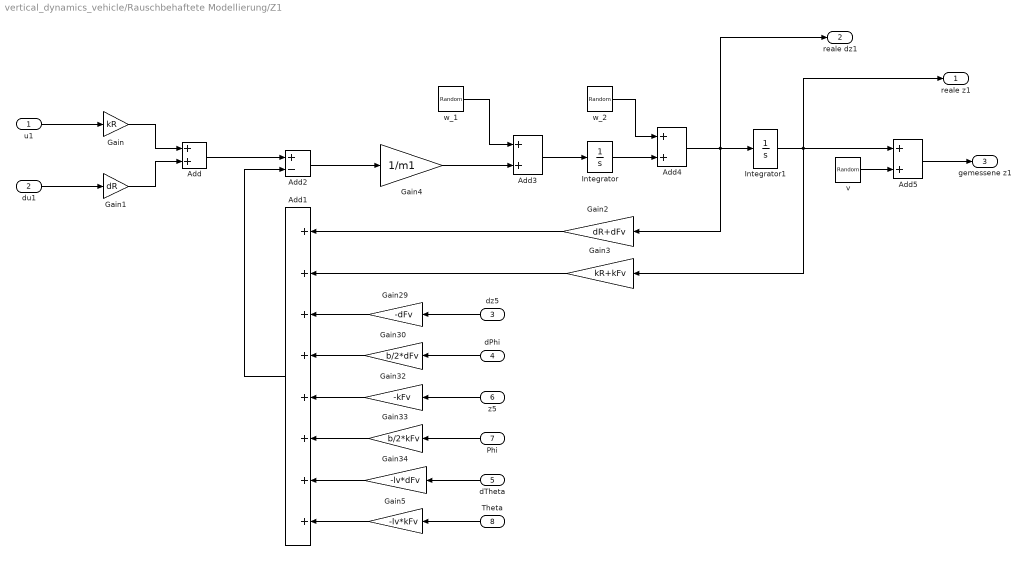
== system vertical_dynamics_vehicle/Rauschbehaftete Modellierung/Z1 ==
  u1 : Inport
  du1 : Inport  Port=2
  dz5 : Inport  Port=3
  dPhi : Inport  Port=4
  dTheta : Inport  Port=5
  z5 : Inport  Port=6
  Phi : Inport  Port=7
  Theta : Inport  Port=8
  Add{,3..5} (4 alike) : Sum
  Add1 : Sum  Inputs=8
  Add2 : Sum  Inputs=+-
  Gain : Gain  Gain=kR
  Gain1 : Gain  Gain=dR
  Gain2 : Gain  Gain=dR+dFv
  Gain29 : Gain  Gain=-dFv
  Gain3 : Gain  Gain=kR+kFv
  Gain30 : Gain  Gain=b/2*dFv
  Gain32 : Gain  Gain=-kFv
  Gain33 : Gain  Gain=b/2*kFv
  Gain34 : Gain  Gain=-lv*dFv
  Gain4 : Gain  Gain=1/m1
  Gain5 : Gain  Gain=-lv*kFv
  Integrator : Integrator  InitialCondition=dz1_0
  Integrator1 : Integrator  InitialCondition=z1_0
  v : RandomNumber  Variance=sigma_mz^2  Seed=seed(3,1)  SampleTime=T_abt
  w_1 : RandomNumber  Variance=sigma_dz^2  Seed=seed(1,1)  SampleTime=T_abt
  w_2 : RandomNumber  Variance=sigma_z^2  Seed=seed(2,1)  SampleTime=T_abt
  reale z1 : Outport
  reale dz1 : Outport  Port=2
  gemessene z1 : Outport  Port=3
  wires:
  Add2/1 -> Gain4/1
  Gain1/1 -> Add/2
  Gain2/1 -> Add1/1
  Add/1 -> Add2/1
  Gain/1 -> Add/1
  Integrator1/1 -> Add5/1, reale z1/1, Gain3/1
  Phi/1 -> Gain33/1
  Gain34/1 -> Add1/7
  Gain32/1 -> Add1/5
  Gain3/1 -> Add1/2
  Gain33/1 -> Add1/6
  u1/1 -> Gain/1
  du1/1 -> Gain1/1
  dTheta/1 -> Gain34/1
  z5/1 -> Gain32/1
  dz5/1 -> Gain29/1
  Gain29/1 -> Add1/3
  Add1/1 -> Add2/2
  Gain30/1 -> Add1/4
  dPhi/1 -> Gain30/1
  Theta/1 -> Gain5/1
  Gain5/1 -> Add1/8
  w_1/1 -> Add3/1
  Gain4/1 -> Add3/2
  Add3/1 -> Integrator/1
  w_2/1 -> Add4/1
  Integrator/1 -> Add4/2
  Add4/1 -> Gain2/1, Integrator1/1, reale dz1/1
  v/1 -> Add5/2
  Add5/1 -> gemessene z1/1

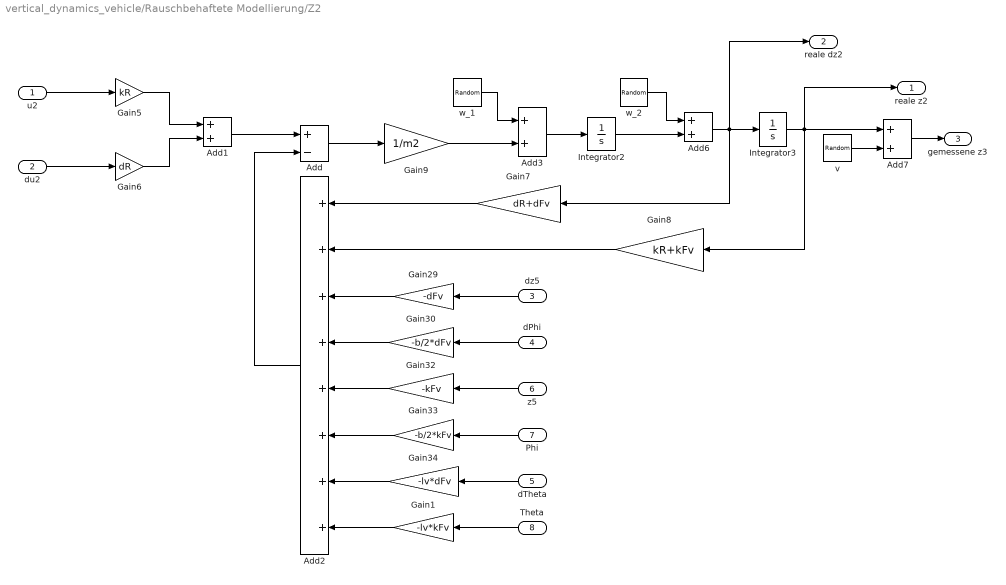
== system vertical_dynamics_vehicle/Rauschbehaftete Modellierung/Z2 ==
  u2 : Inport
  du2 : Inport  Port=2
  dz5 : Inport  Port=3
  dPhi : Inport  Port=4
  dTheta : Inport  Port=5
  z5 : Inport  Port=6
  Phi : Inport  Port=7
  Theta : Inport  Port=8
  Add : Sum  Inputs=+-
  Add{1,3,6..7} (4 alike) : Sum
  Add2 : Sum  Inputs=8
  Gain1 : Gain  Gain=-lv*kFv
  Gain29 : Gain  Gain=-dFv
  Gain30 : Gain  Gain=-b/2*dFv
  Gain32 : Gain  Gain=-kFv
  Gain33 : Gain  Gain=-b/2*kFv
  Gain34 : Gain  Gain=-lv*dFv
  Gain5 : Gain  Gain=kR
  Gain6 : Gain  Gain=dR
  Gain7 : Gain  Gain=dR+dFv
  Gain8 : Gain  Gain=kR+kFv
  Gain9 : Gain  Gain=1/m2
  Integrator2 : Integrator  InitialCondition=dz2_0
  Integrator3 : Integrator  InitialCondition=z2_0
  v : RandomNumber  Variance=sigma_mz^2  Seed=seed(3,1)  SampleTime=T_abt
  w_1 : RandomNumber  Variance=sigma_dz^2  Seed=seed(1,1)  SampleTime=T_abt
  w_2 : RandomNumber  Variance=sigma_z^2  Seed=seed(2,1)  SampleTime=T_abt
  reale z2 : Outport
  reale dz2 : Outport  Port=2
  gemessene z3 : Outport  Port=3
  wires:
  Integrator2/1 -> Add6/2
  Gain5/1 -> Add1/1
  du2/1 -> Gain6/1
  Integrator3/1 -> Gain8/1, Add7/1, reale z2/1
  u2/1 -> Gain5/1
  Gain6/1 -> Add1/2
  Gain30/1 -> Add2/4
  Gain1/1 -> Add2/8
  Theta/1 -> Gain1/1
  dPhi/1 -> Gain30/1
  Gain29/1 -> Add2/3
  Gain8/1 -> Add2/2
  Gain34/1 -> Add2/7
  dz5/1 -> Gain29/1
  Add2/1 -> Add/2
  dTheta/1 -> Gain34/1
  Gain32/1 -> Add2/5
  z5/1 -> Gain32/1
  Gain33/1 -> Add2/6
  Gain7/1 -> Add2/1
  Phi/1 -> Gain33/1
  Add1/1 -> Add/1
  Add/1 -> Gain9/1
  w_1/1 -> Add3/1
  w_2/1 -> Add6/1
  Gain9/1 -> Add3/2
  Add3/1 -> Integrator2/1
  Add6/1 -> Gain7/1, reale dz2/1, Integrator3/1
  v/1 -> Add7/2
  Add7/1 -> gemessene z3/1

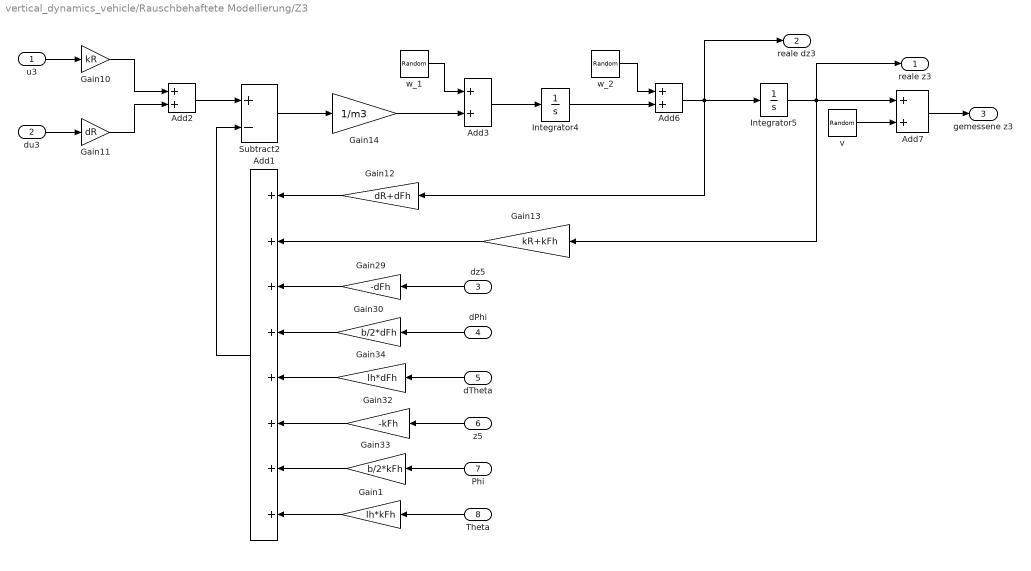
== system vertical_dynamics_vehicle/Rauschbehaftete Modellierung/Z3 ==
  u3 : Inport
  du3 : Inport  Port=2
  dz5 : Inport  Port=3
  dPhi : Inport  Port=4
  dTheta : Inport  Port=5
  z5 : Inport  Port=6
  Phi : Inport  Port=7
  Theta : Inport  Port=8
  Add1 : Sum  Inputs=8
  Add{2..3,6..7} (4 alike) : Sum
  Gain1 : Gain  Gain=lh*kFh
  Gain10 : Gain  Gain=kR
  Gain11 : Gain  Gain=dR
  Gain12 : Gain  Gain=dR+dFh
  Gain13 : Gain  Gain=kR+kFh
  Gain14 : Gain  Gain=1/m3
  Gain29 : Gain  Gain=-dFh
  Gain30 : Gain  Gain=b/2*dFh
  Gain32 : Gain  Gain=-kFh
  Gain33 : Gain  Gain=b/2*kFh
  Gain34 : Gain  Gain=lh*dFh
  Integrator4 : Integrator  InitialCondition=dz3_0
  Integrator5 : Integrator  InitialCondition=z3_0
  Subtract2 : Sum  Inputs=+-
  v : RandomNumber  Variance=sigma_mz^2  Seed=seed(3,1)  SampleTime=T_abt
  w_1 : RandomNumber  Variance=sigma_dz^2  Seed=seed(1,1)  SampleTime=T_abt
  w_2 : RandomNumber  Variance=sigma_z^2  Seed=seed(2,1)  SampleTime=T_abt
  reale z3 : Outport
  reale dz3 : Outport  Port=2
  gemessene z3 : Outport  Port=3
  wires:
  Gain10/1 -> Add2/1
  Add2/1 -> Subtract2/1
  Integrator5/1 -> Add7/1, reale z3/1, Gain13/1
  Gain11/1 -> Add2/2
  Subtract2/1 -> Gain14/1
  du3/1 -> Gain11/1
  u3/1 -> Gain10/1
  Add1/1 -> Subtract2/2
  Gain34/1 -> Add1/5
  Gain32/1 -> Add1/6
  dz5/1 -> Gain29/1
  dPhi/1 -> Gain30/1
  Theta/1 -> Gain1/1
  Gain29/1 -> Add1/3
  Gain30/1 -> Add1/4
  Gain33/1 -> Add1/7
  Gain1/1 -> Add1/8
  Gain12/1 -> Add1/1
  Gain13/1 -> Add1/2
  Phi/1 -> Gain33/1
  z5/1 -> Gain32/1
  dTheta/1 -> Gain34/1
  w_2/1 -> Add6/1
  w_1/1 -> Add3/1
  Gain14/1 -> Add3/2
  Add3/1 -> Integrator4/1
  Integrator4/1 -> Add6/2
  Add6/1 -> reale dz3/1, Integrator5/1, Gain12/1
  v/1 -> Add7/2
  Add7/1 -> gemessene z3/1

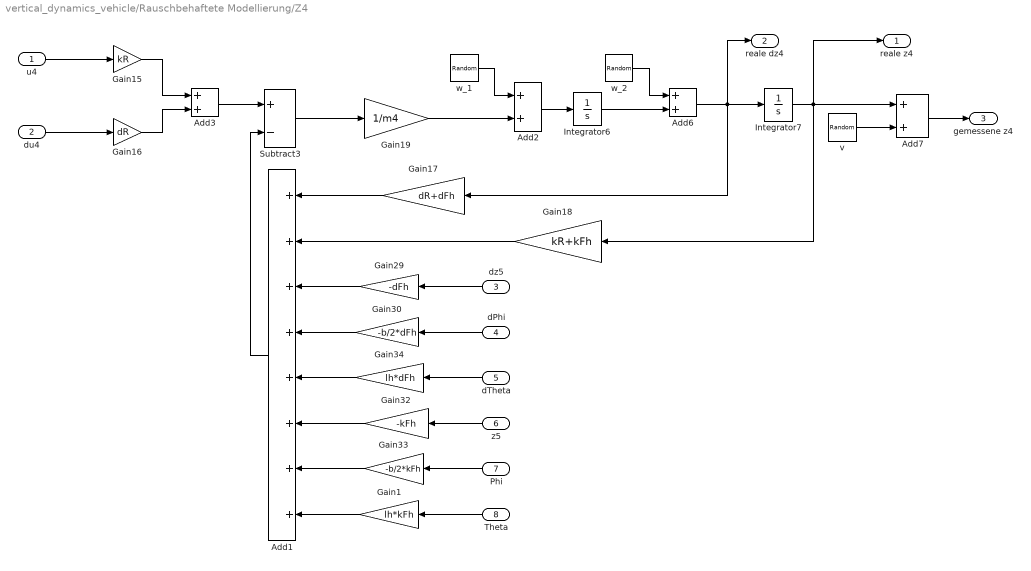
== system vertical_dynamics_vehicle/Rauschbehaftete Modellierung/Z4 ==
  u4 : Inport
  du4 : Inport  Port=2
  dz5 : Inport  Port=3
  dPhi : Inport  Port=4
  dTheta : Inport  Port=5
  z5 : Inport  Port=6
  Phi : Inport  Port=7
  Theta : Inport  Port=8
  Add1 : Sum  Inputs=8
  Add{2..3,6..7} (4 alike) : Sum
  Gain1 : Gain  Gain=lh*kFh
  Gain15 : Gain  Gain=kR
  Gain16 : Gain  Gain=dR
  Gain17 : Gain  Gain=dR+dFh
  Gain18 : Gain  Gain=kR+kFh
  Gain19 : Gain  Gain=1/m4
  Gain29 : Gain  Gain=-dFh
  Gain30 : Gain  Gain=-b/2*dFh
  Gain32 : Gain  Gain=-kFh
  Gain33 : Gain  Gain=-b/2*kFh
  Gain34 : Gain  Gain=lh*dFh
  Integrator6 : Integrator  InitialCondition=dz4_0
  Integrator7 : Integrator  InitialCondition=z4_0
  Subtract3 : Sum  Inputs=+-
  v : RandomNumber  Variance=sigma_mz^2  Seed=seed(3,1)  SampleTime=T_abt
  w_1 : RandomNumber  Variance=sigma_dz^2  Seed=seed(1,1)  SampleTime=T_abt
  w_2 : RandomNumber  Variance=sigma_z^2  Seed=seed(2,1)  SampleTime=T_abt
  reale z4 : Outport
  reale dz4 : Outport  Port=2
  gemessene z4 : Outport  Port=3
  wires:
  Gain16/1 -> Add3/2
  Gain17/1 -> Add1/1
  Gain15/1 -> Add3/1
  Gain19/1 -> Add2/2
  Add3/1 -> Subtract3/1
  Integrator7/1 -> Gain18/1, reale z4/1, Add7/1
  Integrator6/1 -> Add6/2
  Subtract3/1 -> Gain19/1
  du4/1 -> Gain16/1
  u4/1 -> Gain15/1
  Add1/1 -> Subtract3/2
  Phi/1 -> Gain33/1
  z5/1 -> Gain32/1
  dTheta/1 -> Gain34/1
  Gain33/1 -> Add1/7
  dz5/1 -> Gain29/1
  Gain32/1 -> Add1/6
  Gain34/1 -> Add1/5
  Gain29/1 -> Add1/3
  Gain1/1 -> Add1/8
  dPhi/1 -> Gain30/1
  Theta/1 -> Gain1/1
  Gain30/1 -> Add1/4
  Gain18/1 -> Add1/2
  w_2/1 -> Add6/1
  w_1/1 -> Add2/1
  Add2/1 -> Integrator6/1
  Add6/1 -> Integrator7/1, reale dz4/1, Gain17/1
  Add7/1 -> gemessene z4/1
  v/1 -> Add7/2

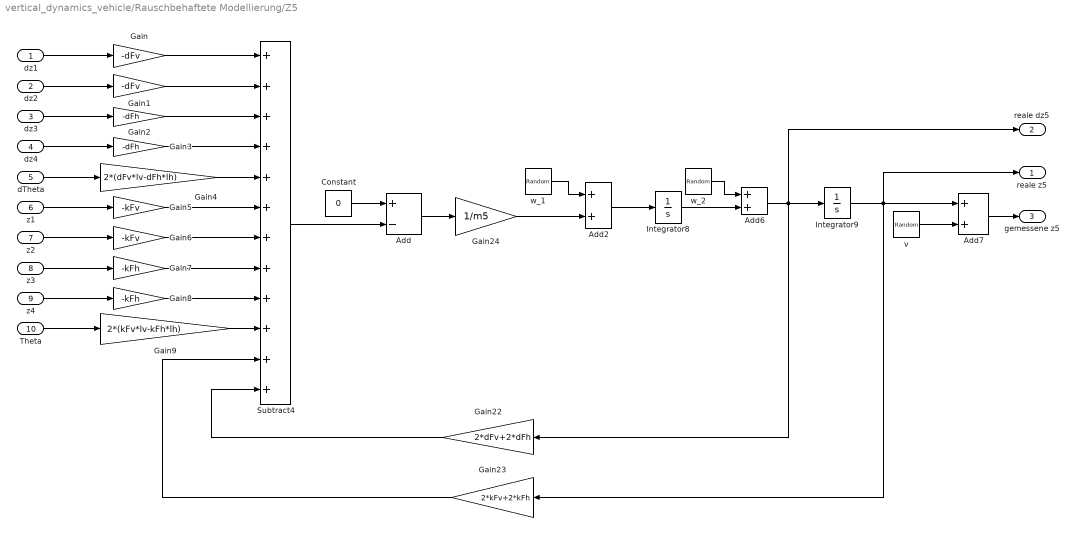
== system vertical_dynamics_vehicle/Rauschbehaftete Modellierung/Z5 ==
  dz1 : Inport
  dz2 : Inport  Port=2
  dz3 : Inport  Port=3
  dz4 : Inport  Port=4
  dTheta : Inport  Port=5
  z1 : Inport  Port=6
  z2 : Inport  Port=7
  z3 : Inport  Port=8
  z4 : Inport  Port=9
  Theta : Inport  Port=10
  Add : Sum  Inputs=+-
  Add2 : Sum
  Add6 : Sum
  Add7 : Sum
  Constant : Constant  Value=0
  Gain : Gain  Gain=-dFv
  Gain1 : Gain  Gain=-dFv
  Gain2 : Gain  Gain=-dFh
  Gain22 : Gain  Gain=2*dFv+2*dFh
  Gain23 : Gain  Gain=2*kFv+2*kFh
  Gain24 : Gain  Gain=1/m5
  Gain3 : Gain  Gain=-dFh
  Gain4 : Gain  Gain=2*(dFv*lv-dFh*lh)
  Gain5 : Gain  Gain=-kFv
  Gain6 : Gain  Gain=-kFv
  Gain7 : Gain  Gain=-kFh
  Gain8 : Gain  Gain=-kFh
  Gain9 : Gain  Gain=2*(kFv*lv-kFh*lh)
  Integrator8 : Integrator  InitialCondition=dz5_0
  Integrator9 : Integrator  InitialCondition=z5_0
  Subtract4 : Sum  Inputs=++++++++++++
  v : RandomNumber  Variance=sigma_mz^2  Seed=seed(3,1)  SampleTime=T_abt
  w_1 : RandomNumber  Variance=sigma_dz^2  Seed=seed(1,1)  SampleTime=T_abt
  w_2 : RandomNumber  Variance=sigma_z^2  Seed=seed(2,1)  SampleTime=T_abt
  reale z5 : Outport
  reale dz5 : Outport  Port=2
  gemessene z5 : Outport  Port=3
  wires:
  Integrator8/1 -> Add6/2
  Subtract4/1 -> Add/2
  dz1/1 -> Gain/1
  Gain/1 -> Subtract4/1
  Gain1/1 -> Subtract4/2
  dz2/1 -> Gain1/1
  dz3/1 -> Gain2/1
  Gain2/1 -> Subtract4/3
  Gain3/1 -> Subtract4/4
  dz4/1 -> Gain3/1
  Gain22/1 -> Subtract4/12
  Gain4/1 -> Subtract4/5
  dTheta/1 -> Gain4/1
  Gain5/1 -> Subtract4/6
  z1/1 -> Gain5/1
  z2/1 -> Gain6/1
  Gain6/1 -> Subtract4/7
  z3/1 -> Gain7/1
  Gain7/1 -> Subtract4/8
  z4/1 -> Gain8/1
  Gain8/1 -> Subtract4/9
  Gain23/1 -> Subtract4/11
  Gain9/1 -> Subtract4/10
  Theta/1 -> Gain9/1
  Add/1 -> Gain24/1
  Constant/1 -> Add/1
  v/1 -> Add7/2
  Add7/1 -> gemessene z5/1
  Integrator9/1 -> Gain23/1, Add7/1, reale z5/1
  w_2/1 -> Add6/1
  w_1/1 -> Add2/1
  Add6/1 -> Gain22/1, Integrator9/1, reale dz5/1
  Add2/1 -> Integrator8/1
  Gain24/1 -> Add2/2
